simulink model "RTW4cycle"  (R2013a)
settings: Solver=ode3  StartTime=0.0  StopTime=inf  FixedStep=0.0025  RelTol=1e-3
undefined symbols (not defined in the file): Serial_Port, Standard_Devices
libraries: rtwinlib x2, simulink x2
settings Model: SimulationMode=external  ExtModeTrigDuration=100000  Creator=ARAS_Robotic1  LastModifiedBy=ARAS_Robotic1
settings HardwareCC: ProdIntDivRoundTo=Zero  ProdEndianess=LittleEndian  ProdHWDeviceType=Generic->32-bit x86 compatible
settings RTWCC: SystemTargetFile=rtwin.tlc  TemplateMakefile=rtwin.tmf  Description=Real-Time Windows Target  ProcessScript=rtwin_make_rtw_hook  RTWCompilerOptimization=On
settings CodeAppCC: MaxIdLength=95
settings RTWinTargetCC: TargetLibSuffix=_rtwin.lib  TargetPreCompLibLocation=C:\Program Files\MATLAB\R2013a\toolbox\rtw\targets\rtwin\lib\win32  CodeReplacementLibrary=ANSI_C  RTWinDir=C:/PROGRA~1/MATLAB/R2013a/toolbox/rtw/targets/rtwin  TargetArch=win32

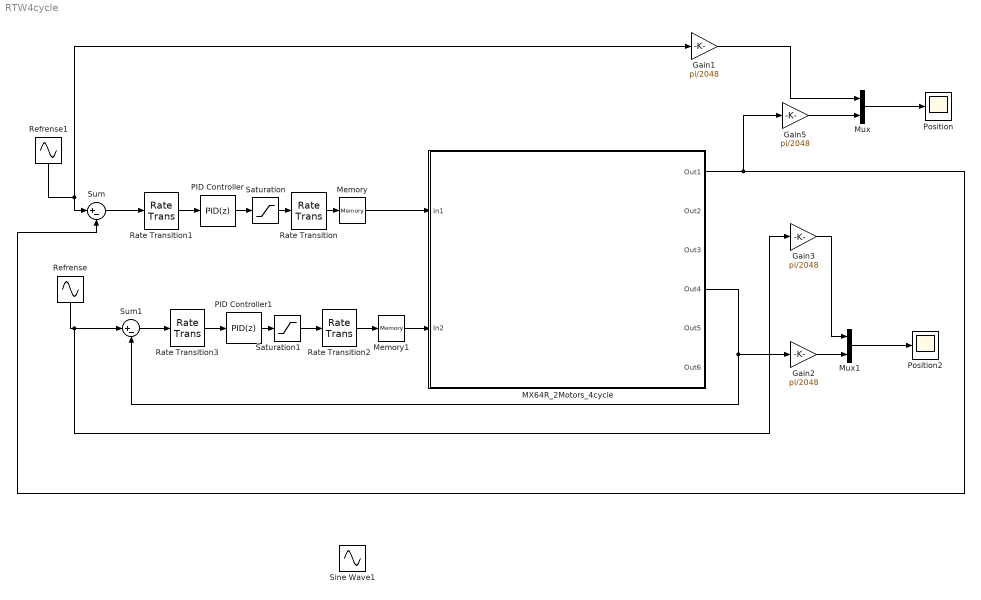
== system RTW4cycle ==
  Gain{1..3,5} (4 alike) : Gain  Gain=pi/2048
  MX64R_2Motors_4cycle : Subsystem  TreatAsAtomicUnit=on  mask(MX64R 2 motors Real Time Windows Target){i1=1, i2=2}
      mask prompts: i1 "ID Dynamixel 1"; i2 "ID Dynamixel 2"
      mask help:
      | This Block is desined for torque control of two Dynamixel motor (MX64R )in real time workshop
      | please be advised with the following issue:
      | Caution1>> change Status Return Level to 1 in EEprom inorder to receive status packet just for read command.
      | Caution2>> It is recommended that Return Delay Time be set as the minimum value within the allowed range of Main Controller.
      | Caution3>> Total sample time for 2 motors is equal to Ts/4. (Ts is the simulink sample time)
      | Copyright @ Aras Lab.
      mask Display:
      | image(imread('mx64RR.jpg'))
      | port_label('input',1,'Torque1')
      | port_label('input',2,'Torque2')
      | port_label('output',1,'position1')
      | port_label('output',2,'velovity1')
      | port_label('output',3,'load1')
      | port_label('output',4,'position2')
      | port_label('output',5,'velovity2')
      | port_label('output',6,'load2')
  Memory : Memory
  Memory1 : Memory
  Mux : Mux  Inputs=2
  Mux1 : Mux  Inputs=2
  PID Controller : simulink/Continuous/PID Controller  Controller=PID  TimeDomain=Discrete-time  SampleTime=0.01  IntegratorMethod=Forward Euler  FilterMethod=Forward Euler  Form=Parallel  P=0.002  I=0.01  D=0.00005  N=100  InitialConditionSource=internal  InitialConditionForIntegrator=0  InitialConditionForFilter=0  ExternalReset=none  LimitOutput=off  UpperSaturationLimit=inf  LowerSaturationLimit=-inf  LinearizeAsGain=on  AntiWindupMode=none  Kb=1  TrackingMode=off  Kt=1  PParamMin=[]  PParamMax=[]  IParamMin=[]  IParamMax=[]  DParamMin=[]  DParamMax=[]  NParamMin=[]  NParamMax=[]  KbParamMin=[]  KbParamMax=[]  KtParamMin=[]  KtParamMax=[]  POutMin=[]  POutMax=[]  IOutMin=[]  IOutMax=[]  DOutMin=[]  DOutMax=[]  NOutMin=[]  NOutMax=[]  KbOutMin=[]  KbOutMax=[]  KtOutMin=[]  KtOutMax=[]  IntegratorOutMin=[]  IntegratorOutMax=[]  FilterOutMin=[]  FilterOutMax=[]  SumOutMin=[]  SumOutMax=[]  SumI1OutMin=[]  SumI1OutMax=[]  SumI2OutMin=[]  SumI2OutMax=[]  SumI3OutMin=[]  SumI3OutMax=[]  SumDOutMin=[]  SumDOutMax=[]  SaturationOutMin=[]  SaturationOutMax=[]  IntegratorContinuousStateAttributes=''  IntegratorStateMustResolveToSignalObject=off  IntegratorRTWStateStorageClass=Auto  FilterContinuousStateAttributes=''  FilterStateMustResolveToSignalObject=off  FilterRTWStateStorageClass=Auto
      link override Filter: IntegratorMethod=Integration: Forward Euler  gainval=1.0  ExternalReset=none  InitialConditionSource=internal  InitialCondition=InitialConditionForFilter  InitialConditionMode=State only (most efficient)  SampleTime=-1  OutMin=FilterOutMin  OutMax=FilterOutMax  OutDataTypeStr=FilterOutDataTypeStr  LimitOutput=off  UpperSaturationLimit=inf  LowerSaturationLimit=-inf  ShowSaturationPort=off  ShowStatePort=off
      link override Filter: StateMustResolveToSignalObject=off  RTWStateStorageClass=Auto
  PID Controller1 : simulink/Continuous/PID Controller  Controller=PID  TimeDomain=Discrete-time  SampleTime=0.01  IntegratorMethod=Forward Euler  FilterMethod=Forward Euler  Form=Parallel  P=0.002  I=0.01  D=0.00005  N=100  InitialConditionSource=internal  InitialConditionForIntegrator=0  InitialConditionForFilter=0  ExternalReset=none  LimitOutput=off  UpperSaturationLimit=inf  LowerSaturationLimit=-inf  LinearizeAsGain=on  AntiWindupMode=none  Kb=1  TrackingMode=off  Kt=1  PParamMin=[]  PParamMax=[]  IParamMin=[]  IParamMax=[]  DParamMin=[]  DParamMax=[]  NParamMin=[]  NParamMax=[]  KbParamMin=[]  KbParamMax=[]  KtParamMin=[]  KtParamMax=[]  POutMin=[]  POutMax=[]  IOutMin=[]  IOutMax=[]  DOutMin=[]  DOutMax=[]  NOutMin=[]  NOutMax=[]  KbOutMin=[]  KbOutMax=[]  KtOutMin=[]  KtOutMax=[]  IntegratorOutMin=[]  IntegratorOutMax=[]  FilterOutMin=[]  FilterOutMax=[]  SumOutMin=[]  SumOutMax=[]  SumI1OutMin=[]  SumI1OutMax=[]  SumI2OutMin=[]  SumI2OutMax=[]  SumI3OutMin=[]  SumI3OutMax=[]  SumDOutMin=[]  SumDOutMax=[]  SaturationOutMin=[]  SaturationOutMax=[]  IntegratorContinuousStateAttributes=''  IntegratorStateMustResolveToSignalObject=off  IntegratorRTWStateStorageClass=Auto  FilterContinuousStateAttributes=''  FilterStateMustResolveToSignalObject=off  FilterRTWStateStorageClass=Auto
      link override Filter: IntegratorMethod=Integration: Forward Euler  gainval=1.0  ExternalReset=none  InitialConditionSource=internal  InitialCondition=InitialConditionForFilter  InitialConditionMode=State only (most efficient)  SampleTime=-1  OutMin=FilterOutMin  OutMax=FilterOutMax  OutDataTypeStr=FilterOutDataTypeStr  LimitOutput=off  UpperSaturationLimit=inf  LowerSaturationLimit=-inf  ShowSaturationPort=off  ShowStatePort=off
      link override Filter: StateMustResolveToSignalObject=off  RTWStateStorageClass=Auto
  Position : Scope
      settings: TimeRange=10  YMin=0  YMax=2500  SaveName=ScopeData6
  Position2 : Scope
      settings: TimeRange=10  YMin=0  YMax=130  SaveName=ScopeData7
  Rate Transition : RateTransition
  Rate Transition1 : RateTransition  OutPortSampleTime=0.01
  Rate Transition2 : RateTransition
  Rate Transition3 : RateTransition  OutPortSampleTime=0.01
  Refrense : Sin  Amplitude=500  Bias=2000  Frequency=1.5
  Refrense1 : Sin  Amplitude=500  Bias=2000  Frequency=1.5
  Saturation : Saturate  UpperLimit=6  LowerLimit=-6
  Saturation1 : Saturate  UpperLimit=6  LowerLimit=-6
  Sine Wave1 : Sin  Amplitude=0.3  Frequency=2
  Sum : Sum  Inputs=|+-
  Sum1 : Sum  Inputs=|+-
  wires:
  Sum/1 -> Rate Transition1/1
  PID Controller/1 -> Saturation/1
  Saturation/1 -> Rate Transition/1
  Rate Transition/1 -> Memory/1
  Rate Transition1/1 -> PID Controller/1
  Mux/1 -> Position/1
  Refrense1/1 -> Sum/1, Gain1/1
  MX64R_2Motors_4cycle/1(Out1) -> Gain5/1, Sum/2
  Gain1/1 -> Mux/1
  Sum1/1 -> Rate Transition3/1
  PID Controller1/1 -> Saturation1/1
  Saturation1/1 -> Rate Transition2/1
  Rate Transition2/1 -> Memory1/1
  Rate Transition3/1 -> PID Controller1/1
  Refrense/1 -> Gain3/1, Sum1/1
  Mux1/1 -> Position2/1
  Gain3/1 -> Mux1/1
  MX64R_2Motors_4cycle/4(Out4) -> Gain2/1, Sum1/2
  Memory/1 -> MX64R_2Motors_4cycle/1(In1)
  Memory1/1 -> MX64R_2Motors_4cycle/2(In2)
  Gain5/1 -> Mux/2
  Gain2/1 -> Mux1/2

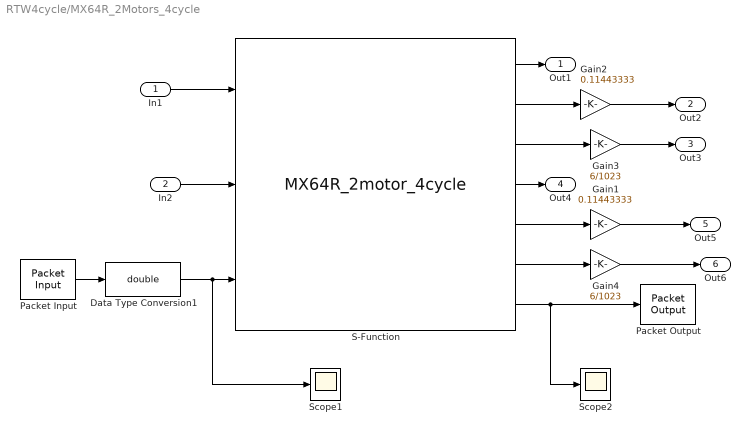
== system RTW4cycle/MX64R_2Motors_4cycle ==
  In1 : Inport
  In2 : Inport  Port=2
  Data Type Conversion1 : DataTypeConversion  OutDataTypeStr=double  ConvertRealWorld=Stored Integer (SI)
  Gain1 : Gain  Gain=0.11443333
  Gain2 : Gain  Gain=0.11443333
  Gain3 : Gain  Gain=6/1023
  Gain4 : Gain  Gain=6/1023
  Packet Input : rtwinlib/Packet Input  SampleTime=-1  MaxMissedTicks=1  ShowMissedTicks=off  YieldWhenWaiting=off  DrvName=Standard_Devices/Serial_Port  DrvAddress=3  DrvOptions=[3000000 8 0 0 0 1 0 0]  PacketSize=12  DataTypes='12*uint8'  ShowReady=off  ShowError=off  PacketID=1  ByteOrder=1  ShowTimestamp=off
      settings: AttributesFormatString=Standard Devices\nSerial Port [3h]
  Packet Output : rtwinlib/Packet Output  SampleTime=-1  MaxMissedTicks=1  ShowMissedTicks=off  YieldWhenWaiting=off  DrvName=Standard_Devices/Serial_Port  DrvAddress=3  DrvOptions=[3000000 8 0 0 0 1 0 0]  PacketSize=10  DataTypes='10*uint8'  ShowReady=off  ShowError=off  PacketID=1  ByteOrder=1  InitialValue=[]  FinalValue=[]
      settings: AttributesFormatString=Standard Devices\nSerial Port [3h]
  S-Function : S-Function  FunctionName=MX64R_2motor_4cycle  Parameters=i1,i2  EnableBusSupport=off
      mask Display:
      | port_label('input',1,'desire torque1')
      | port_label('input',2,'desire torque2')
      | port_label('input',3,'serial in')
      | port_label('output',1,'position1')
      | port_label('output',2,'velocity1')
      | port_label('output',3,'load1')
      | port_label('output',4,'position2')
      | port_label('output',5,'velocity2')
      | port_label('output',6,'load2')
      | port_label('output',7,'serial out')
  Scope1 : Scope
      settings: TimeRange=10  YMin=0  YMax=275
  Scope2 : Scope
      settings: TimeRange=10  YMin=0  YMax=275
  Out1 : Outport
  Out2 : Outport  Port=2
  Out3 : Outport  Port=3
  Out4 : Outport  Port=4
  Out5 : Outport  Port=5
  Out6 : Outport  Port=6
  wires:
  S-Function/7 -> Scope2/1, Packet Output/1
  Packet Input/1 -> Data Type Conversion1/1
  Data Type Conversion1/1 -> Scope1/1, S-Function/3
  In1/1 -> S-Function/1
  S-Function/1 -> Out1/1
  S-Function/2 -> Gain2/1
  In2/1 -> S-Function/2
  S-Function/4 -> Out4/1
  S-Function/3 -> Gain3/1
  S-Function/5 -> Gain1/1
  S-Function/6 -> Gain4/1
  Gain2/1 -> Out2/1
  Gain1/1 -> Out5/1
  Gain3/1 -> Out3/1
  Gain4/1 -> Out6/1
